simulink model "C01_1"  (R2021a)
settings: Solver=VariableStepAuto  StartTime=0.0  StopTime=10.0  RelTol=1e-3
libraries: simulink x2
settings Model: Creator=riobe  LastModifiedBy=riobe

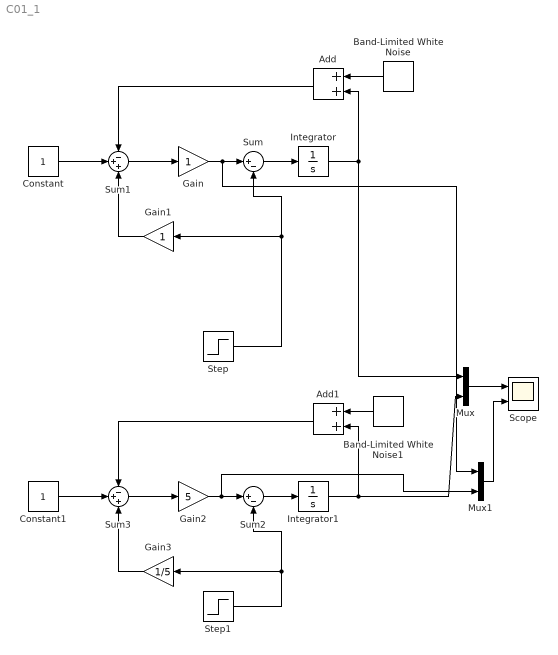
== system C01_1 ==
  Add : Sum
  Add1 : Sum
  Band-Limited White Noise : simulink/Sources/Band-Limited White Noise  Cov=[0.001]  Ts=0.1  seed=[23341]
  Band-Limited White Noise1 : simulink/Sources/Band-Limited White Noise  Cov=[0.001]  Ts=0.1  seed=[23341]
  Constant : Constant
  Constant1 : Constant
  Gain : Gain
  Gain1 : Gain
  Gain2 : Gain  Gain=5
  Gain3 : Gain  Gain=1/5
  Integrator : Integrator
  Integrator1 : Integrator
  Mux : Mux  Inputs=2
  Mux1 : Mux  Inputs=2
  Scope : Scope  NumInputPorts=2
  Step : Step  Before=0.5  After=0.8  SampleTime=0
  Step1 : Step  Before=0.5  After=0.8  SampleTime=0
  Sum : Sum  Inputs=|+-
  Sum1 : Sum  Inputs=-++
  Sum2 : Sum  Inputs=|+-
  Sum3 : Sum  Inputs=-++
  wires:
  Sum/1 -> Integrator/1
  Gain/1 -> Mux1/1, Sum/1
  Sum1/1 -> Gain/1
  Step/1 -> Gain1/1, Sum/2
  Constant/1 -> Sum1/2
  Add/1 -> Sum1/1
  Integrator/1 -> Add/2, Mux/1
  Integrator1/1 -> Add1/2, Mux/2
  Add1/1 -> Sum3/1
  Constant1/1 -> Sum3/2
  Step1/1 -> Sum2/2, Gain3/1
  Sum3/1 -> Gain2/1
  Gain2/1 -> Mux1/2, Sum2/1
  Sum2/1 -> Integrator1/1
  Mux/1 -> Scope/1
  Mux1/1 -> Scope/2
  Gain3/1 -> Sum3/3
  Gain1/1 -> Sum1/3
  Band-Limited White Noise/1 -> Add/1
  Band-Limited White Noise1/1 -> Add1/1
